simulink model "bldc_speed_control"  (R2020a)
settings: Solver=ode45  StartTime=0.0  StopTime=10  RelTol=1e-3
libraries: simulink_extras x2
settings Model: Creator=HP  LastModifiedBy=INDRAJIT MARATHE

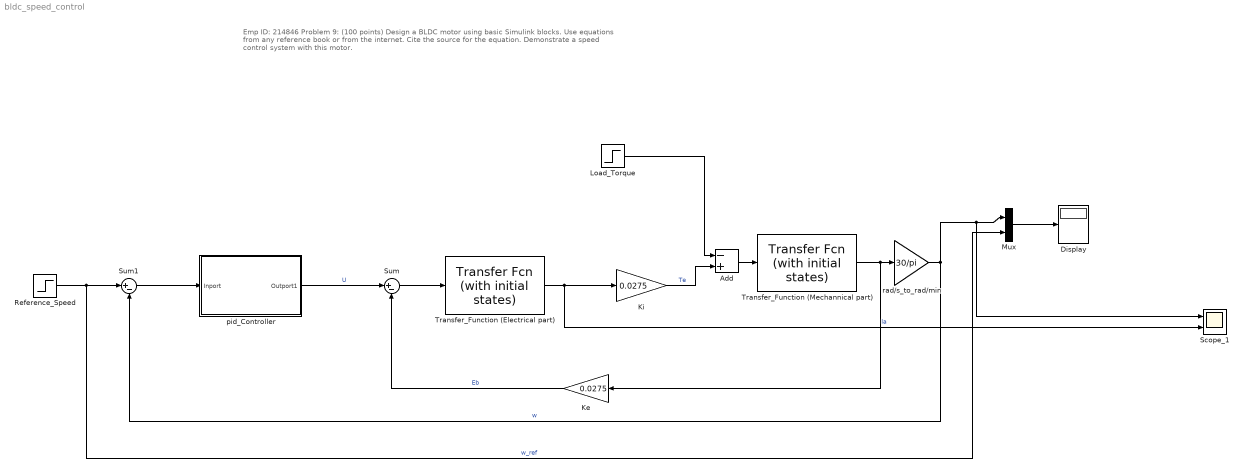
== system bldc_speed_control ==
  note: Emp ID: 214846
      |
      | Problem 9: (100 points) Design a BLDC motor using basic Simulink blocks.
      | Use equations from any reference book or from the internet.
      | Cite the source for the equation.
      | Demonstrate a speed control system with this motor.
  Add : Sum  Inputs=-+
  Display : Display
  Ke : Gain  Gain=0.0275
  Ki : Gain  Gain=0.0275
  Load_Torque : Step  Time=0.1  After=10  SampleTime=0
  Mux : Mux  Inputs=2
  Reference_Speed : Step  After=50  SampleTime=0
  Scope_1 : Scope  NumInputPorts=2
  Sum : Sum  Inputs=|+-
  Sum1 : Sum  Inputs=|+-
  Transfer_Function (Electrical part) : simulink_extras/Additional Linear/Transfer Fcn (with initial states)  N=[1]  D="[0.0001  0.014]"  X0=.5
  Transfer_Function (Mechannical part) : simulink_extras/Additional Linear/Transfer Fcn (with initial states)  N=[1]  D="[0.0002  0.004586]"  X0=.5
  pid_Controller : Subsystem
  rad/s_to_rad/min : Gain  Gain=30/pi
  wires:
  Ke/1 -> Sum/2  "Eb"
  pid_Controller/1(Outport1) -> Sum/1  "U"
  Sum1/1 -> pid_Controller/1(Inport)
  Sum/1 -> Transfer_Function (Electrical part)/1
  Transfer_Function (Electrical part)/1 -> Scope_1/2, Ki/1  "la"
  Ki/1 -> Add/2  "Te"
  Add/1 -> Transfer_Function (Mechannical part)/1
  Load_Torque/1 -> Add/1
  Transfer_Function (Mechannical part)/1 -> rad/s_to_rad/min/1, Ke/1
  Reference_Speed/1 -> Mux/2, Sum1/1  "w_ref"
  rad/s_to_rad/min/1 -> Scope_1/1, Mux/1, Sum1/2  "w"
  Mux/1 -> Display/1

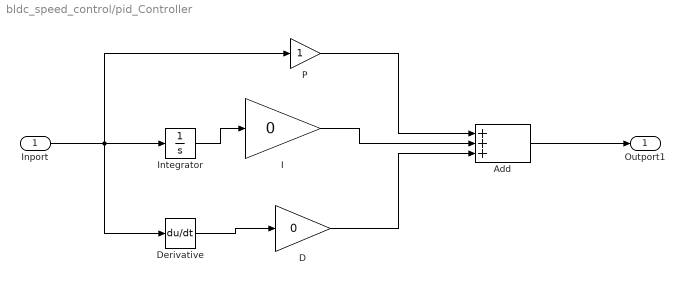
== system bldc_speed_control/pid_Controller ==
  Inport : Inport
  Add : Sum  Inputs=+++
  D : Gain  Gain=0
  Derivative : Derivative
  I : Gain  Gain=0
  Integrator : Integrator
  P : Gain
  Outport1 : Outport
  wires:
  Add/1 -> Outport1/1
  Inport/1 -> P/1, Derivative/1, Integrator/1
  Integrator/1 -> I/1
  I/1 -> Add/2
  D/1 -> Add/3
  P/1 -> Add/1
  Derivative/1 -> D/1
